simulink model "INS"  (R2022b)
settings: configuration reference "ins_config" (kept outside this file)
values from neighbouring files (symbols this model uses):
  INS_EXPORT = Simulink.Parameter(INS_EXPORT_VALUE)    [ins_model_init.m]
  INS_PARAM = Simulink.Parameter(INS_PARAM_VALUE)    [ins_model_init.m]
undefined symbols (not defined in the file or in its folder): DiscIntNeverNeededParam, INS_CONST, INS_EXPORT_VALUE
libraries: simulink x116, FMT_Model_Lib x35
(part 5 of 5)

== system INS/Data_Fusion/Rotation_Filter/AHRS/Correct/Attitude_Correction/Attitude_Correct/Acc_Estimator/Measure_Acc/GPS_Meas_Acc ==
  reset : Inport
  gps_vel_O_mPs : Inport  Port=2
  Enable : EnablePort  StatesWhenEnabling=reset
  Integrator : DiscreteIntegrator  ExternalReset=level  SampleTime=-1  ICPrevOutput=DiscIntNeverNeededParam  ICPrevScaledInput=DiscIntNeverNeededParam
  Integrator1 : DiscreteIntegrator  ExternalReset=level  InitialConditionSource=external  SampleTime=-1  ICPrevOutput=DiscIntNeverNeededParam  ICPrevScaledInput=DiscIntNeverNeededParam
  Sum : Sum  Inputs=|++
  Sum1 : Sum  Inputs=|+-
  gain : Gain  Gain=2*zeta*fc
  gain1 : Gain  Gain=fc^2
  gps_acc_O_mPs2 : Outport  VectorParamsAs1DForOutWhenUnconnected=off
  wires:
  Integrator1/1 -> Sum1/2
  Integrator/1 -> gps_acc_O_mPs2/1, Sum/2
  reset/1 -> Integrator1/2, Integrator/2
  gain/1 -> Sum/1
  Sum1/1 -> gain/1, gain1/1
  Sum/1 -> Integrator1/1
  gps_vel_O_mPs/1 -> Sum1/1, Integrator1/3
  gain1/1 -> Integrator/1

== system INS/Data_Fusion/Rotation_Filter/AHRS/Correct/Attitude_Correction/Attitude_Correct/Acc_Estimator/Measure_Acc/Valid_Check ==
  Sensor_Data : Inport
  Bus Selector : BusSelector  OutputSignals=GPS_Data.GPS_valid,GPS_Data.spd_quality
  Logical Operator1 : Logic  AllPortsSameDT=off  OutDataTypeStr=boolean
  Relay : Relay  OnSwitchValue=0.2  OffSwitchValue=0.1
  gps_meas_acc_valid : Outport  VectorParamsAs1DForOutWhenUnconnected=off
  wires:
  Sensor_Data/1 -> Bus Selector/1
  Logical Operator1/1 -> gps_meas_acc_valid/1
  Bus Selector/1 -> Logical Operator1/1  "<GPS_valid>"
  Relay/1 -> Logical Operator1/2
  Bus Selector/2 -> Relay/1  "<spd_quality>"

== system INS/Data_Fusion/Translation_Filter/CF/Bus_Constructor/Bus_Select/WGS84_Position/WGS84_Position/safe_divide/Zero_Value_Exclusion ==
  u : Inport
  Abs : Abs  SaturateOnIntegerOverflow=off
  Constant : Constant
  Product : Product  RndMeth=Zero
  Saturation : Saturate  UpperLimit=10e7  LowerLimit=1e-6
  Sign : Signum
  Switch : Switch  Criteria=u2 ~= 0  SaturateOnIntegerOverflow=off  InputSameDT=off
  y : Outport  VectorParamsAs1DForOutWhenUnconnected=off
  wires:
  u/1 -> Abs/1, Sign/1
  Abs/1 -> Saturation/1
  Saturation/1 -> Product/1
  Sign/1 -> Switch/2, Switch/1
  Product/1 -> y/1
  Switch/1 -> Product/2
  Constant/1 -> Switch/3

== system INS/Data_Fusion/Translation_Filter/CF/Horizontal_Filter/Correct/GPS Correct/GPS_Correct/Measurement/Bias_Estimation ==
  TF_Data : Inport
  X : Inport  Port=2
  xy_meas_m : Inport  Port=3
  Bias : Subsystem
  Sum1 : Sum  Inputs=|++
  bias_update : Outport  VectorParamsAs1DForOutWhenUnconnected=off
  xy_O_m : Outport  Port=2  VectorParamsAs1DForOutWhenUnconnected=off
  wires:
  TF_Data/1 -> Bias/3(TF_Data)
  X/1 -> Bias/2(X)
  Sum1/1 -> xy_O_m/1
  Bias/1(bias) -> Sum1/2
  xy_meas_m/1 -> Sum1/1, Bias/1(xy_meas_m)  "gps_xy_m"
  Bias/2(bias_update) -> bias_update/1

== system INS/Data_Fusion/Translation_Filter/CF/Horizontal_Filter/Predict/Propagate/States_Init/Pos_Init/GPS_Pos_Init ==
  TF_Data : Inport
  Enable : EnablePort
  Bus Selector : BusSelector  OutputSignals=Sensor_Meas.GPS_Meas.lat_rad,Sensor_Meas.GPS_Meas.lon_rad,TF_Control.WGS84_Ref.WGS84_pos_ref.lat_0_rad,TF_Control.WGS84_Ref.WGS84_pos_ref.lon_0_rad,TF_Control.WGS84_Ref.WGS84_derivatives_ref.dx_dlat_0,TF_Control.WGS84_Ref.WGS84_derivatives_ref.dy_dlon_0
  Data Type Conversion : DataTypeConversion  OutDataTypeStr=single  SaturateOnIntegerOverflow=off  RndMeth=Floor
  Multiply : Product
  Mux1 : Mux  Inputs=2
  Mux2 : Mux  Inputs=2
  Mux3 : Mux  Inputs=2
  Sum : Sum  Inputs=|+-
  X_0 : Outport  VectorParamsAs1DForOutWhenUnconnected=off
  wires:
  Data Type Conversion/1 -> X_0/1
  Bus Selector/1 -> Mux1/1  "<lat_rad>"
  Mux3/1 -> Multiply/2
  Bus Selector/3 -> Mux2/1  "<lat_0_rad>"
  Bus Selector/4 -> Mux2/2  "<lon_0_rad>"
  Mux2/1 -> Sum/2
  Bus Selector/6 -> Mux3/2  "<dy_dlon_0>"
  Mux1/1 -> Sum/1
  Sum/1 -> Multiply/1
  Bus Selector/5 -> Mux3/1  "<dx_dlat_0>"
  Bus Selector/2 -> Mux1/2  "<lon_rad>"
  TF_Data/1 -> Bus Selector/1
  Multiply/1 -> Data Type Conversion/1  "xy_R_m"

== system INS/Data_Fusion/Translation_Filter/CF/Horizontal_Filter/Predict/Propagate/States_Init/Vel_Init/GPS_Vel_Init ==
  Processed_Data : Inport
  Enable : EnablePort
  Bus Selector : BusSelector  OutputSignals=Sensor_Meas.GPS_Meas.vn_mPs,Sensor_Meas.GPS_Meas.ve_mPs
  Mux : Mux  Inputs=2
  Reshape : Reshape  OutputDimensionality=Customize  OutputDimensions=[2,1]
  Vel_NE_0 : Outport  VectorParamsAs1DForOutWhenUnconnected=off
  wires:
  Mux/1 -> Reshape/1
  Reshape/1 -> Vel_NE_0/1
  Bus Selector/2 -> Mux/2  "<ve_mPs>"
  Bus Selector/1 -> Mux/1  "<vn_mPs>"
  Processed_Data/1 -> Bus Selector/1

== system INS/Data_Fusion/Translation_Filter/CF/Horizontal_Filter/Predict/Propagate/States_Init/Vel_Init/OptFlow_Vel_Init ==
  Processed_Data : Inport
  Enable : EnablePort
  Bus Selector : BusSelector  OutputSignals=Sensor_Meas.OptFlow_Meas.vx_O_mPs,Sensor_Meas.OptFlow_Meas.vy_O_mPs
  Mux : Mux  Inputs=2
  Reshape : Reshape  OutputDimensionality=Column vector (2-D)  OutputDimensions=[2,1]
  Vel_NE_0 : Outport  VectorParamsAs1DForOutWhenUnconnected=off
  wires:
  Processed_Data/1 -> Bus Selector/1
  Bus Selector/1 -> Mux/1  "<vx_O_mPs>"
  Bus Selector/2 -> Mux/2  "<vy_O_mPs>"
  Reshape/1 -> Vel_NE_0/1
  Mux/1 -> Reshape/1

== system INS/Data_Fusion/Translation_Filter/CF/Verticle_Filter/Correct/Baro_Correct/Baro_Correct/Measurement/Bias_Estimation ==
  h_m : Inport
  TF_Data : Inport  Port=2
  X : Inport  Port=3
  Bias : Subsystem
  Bus Selector1 : BusSelector  OutputSignals=Sensor_Enable.vert_select.baro_enable
  Delay : Delay  DelayLength=1
  Detect Increase : simulink/Logic and Bit Operations/Detect Increase  vinit=0  OutDataTypeStr=boolean
  Selector : Selector  InputPortWidth=3  IndexOptions=Index vector (dialog)  Indices=1  OutputSizes=1
  Switch : Switch  Criteria=u2 > Threshold  OutDataTypeStr=single  SaturateOnIntegerOverflow=off  InputSameDT=off
  bias : Outport  VectorParamsAs1DForOutWhenUnconnected=off
  bias_update : Outport  Port=2  VectorParamsAs1DForOutWhenUnconnected=off
  wires:
  Delay/1 -> Switch/3
  X/1 -> Selector/1
  Bias/1(bias) -> Switch/1
  Switch/1 -> Delay/1, bias/1  "baro_alt_bias"
  Selector/1 -> Bias/1(height_est_m)
  h_m/1 -> Bias/2(height_meas_m)
  Bus Selector1/1 -> Detect Increase/1  "<baro_enable>"
  TF_Data/1 -> Bus Selector1/1
  Detect Increase/1 -> bias_update/1, Switch/2  "baro_bias_update"

== system INS/Data_Fusion/Translation_Filter/CF/Verticle_Filter/Correct/GPS_Correct/GPS_Correct/Measurement/Bias_Estimation ==
  h_m : Inport
  X : Inport  Port=2
  TF_Data : Inport  Port=3
  Bias : Subsystem
  Bus Selector1 : BusSelector  OutputSignals=Sensor_Enable.vert_select.gps_enable
  Detect Increase : simulink/Logic and Bit Operations/Detect Increase  vinit=0.0  OutDataTypeStr=boolean
  Memory : Memory
  Selector : Selector  InputPortWidth=3  IndexOptions=Index vector (dialog)  Indices=1  OutputSizes=1
  Switch : Switch  Criteria=u2 > Threshold  OutDataTypeStr=single  SaturateOnIntegerOverflow=off  InputSameDT=off
  bias : Outport  VectorParamsAs1DForOutWhenUnconnected=off
  bias_update : Outport  Port=2  VectorParamsAs1DForOutWhenUnconnected=off
  wires:
  Memory/1 -> Switch/3
  X/1 -> Selector/1
  Bias/1(bias) -> Switch/1
  Switch/1 -> Memory/1, bias/1  "gps_height_bias"
  Selector/1 -> Bias/1(h_est_m)  "h_est_m1"
  Bus Selector1/1 -> Detect Increase/1  "<gps_enable>"
  Detect Increase/1 -> bias_update/1, Switch/2
  TF_Data/1 -> Bus Selector1/1
  h_m/1 -> Bias/2(h_meas_m)  "gps_h_meas"

== system INS/Data_Fusion/Translation_Filter/CF/Verticle_Filter/Correct/Rf_Correct/Rangefinder_Correct/Measurement/Bias_Estimation ==
  h_m : Inport
  X : Inport  Port=2
  TF_Data : Inport  Port=3
  Bias : Subsystem
  Bus Selector1 : BusSelector  OutputSignals=Sensor_Enable.vert_select.rf_enable
  Detect Increase : simulink/Logic and Bit Operations/Detect Increase  vinit=0.0  OutDataTypeStr=boolean
  Detect_Jump_Signal : Subsystem
  Logical Operator : Logic  Operator=OR  AllPortsSameDT=off  OutDataTypeStr=boolean
  Memory : Memory
  Selector : Selector  InputPortWidth=3  IndexOptions=Index vector (dialog)  Indices=1  OutputSizes=1
  Switch : Switch  Criteria=u2 > Threshold  OutDataTypeStr=single  SaturateOnIntegerOverflow=off  InputSameDT=off
  bias : Outport  VectorParamsAs1DForOutWhenUnconnected=off
  bias_update : Outport  Port=2  VectorParamsAs1DForOutWhenUnconnected=off
  wires:
  Memory/1 -> Switch/3
  X/1 -> Selector/1
  Bias/1(bias) -> Switch/1
  Switch/1 -> Memory/1, bias/1  "rf_height_bias"
  Selector/1 -> Bias/1(h_est_m)  "rf_h_est_m"
  Bus Selector1/1 -> Detect Increase/1  "<rf_enable>"
  Logical Operator/1 -> Switch/2, bias_update/1
  TF_Data/1 -> Bus Selector1/1
  h_m/1 -> Detect_Jump_Signal/1(h_meas_m), Bias/2(h_meas_m)  "rf_h_meas"
  Detect Increase/1 -> Logical Operator/1
  Detect_Jump_Signal/1(update) -> Logical Operator/2

== system INS/Data_Fusion/Translation_Filter/CF/Verticle_Filter/Predict/Propagate/States_Init/Height_Init/Baro_Reference_Height ==
  TF_Data : Inport
  Enable : EnablePort
  Bus Selector : BusSelector  OutputSignals=Sensor_Meas.Baro_Meas.h_R_m
  Data Type Conversion : DataTypeConversion  OutDataTypeStr=single  SaturateOnIntegerOverflow=off  RndMeth=Floor
  h_R_m : Outport  VectorParamsAs1DForOutWhenUnconnected=off
  wires:
  Data Type Conversion/1 -> h_R_m/1
  Bus Selector/1 -> Data Type Conversion/1  "<h_R_m>"
  TF_Data/1 -> Bus Selector/1

== system INS/Data_Fusion/Translation_Filter/CF/Verticle_Filter/Predict/Propagate/States_Init/Height_Init/GPS_Reference_Height ==
  TF_Data : Inport
  Enable : EnablePort
  Bus Selector : BusSelector  OutputSignals=Sensor_Meas.GPS_Meas.h_m,TF_Control.WGS84_Ref.WGS84_pos_ref.h_0_m
  Data Type Conversion : DataTypeConversion  OutDataTypeStr=single  SaturateOnIntegerOverflow=off  RndMeth=Floor
  Sum : Sum  Inputs=|+-
  h_R_m : Outport  VectorParamsAs1DForOutWhenUnconnected=off
  wires:
  Data Type Conversion/1 -> h_R_m/1
  Bus Selector/2 -> Sum/2  "<h_0_m>"
  Bus Selector/1 -> Sum/1  "<h_m>"
  TF_Data/1 -> Bus Selector/1
  Sum/1 -> Data Type Conversion/1  "h_R_m"

== system INS/Data_Fusion/Translation_Filter/CF/Verticle_Filter/Predict/Propagate/States_Init/Height_Init/Rf_Reference_Height ==
  TF_Data : Inport
  Enable : EnablePort
  Bus Selector : BusSelector  OutputSignals=Sensor_Meas.Rf_Meas.h_AGL_m
  Data Type Conversion : DataTypeConversion  OutDataTypeStr=single  SaturateOnIntegerOverflow=off  RndMeth=Floor
  h_R_m : Outport  VectorParamsAs1DForOutWhenUnconnected=off
  wires:
  TF_Data/1 -> Bus Selector/1
  Bus Selector/1 -> Data Type Conversion/1  "<h_AGL_m>"
  Data Type Conversion/1 -> h_R_m/1

== system INS/Data_Fusion/Translation_Filter/CF/Verticle_Filter/Predict/Propagate/States_Init/Velocity_Init/Baro_Velocity ==
  TF_Data : Inport
  Enable : EnablePort
  Constant : Constant  Value=0  OutDataTypeStr=single
  Terminator : Terminator
  vel_D_mPs : Outport  VectorParamsAs1DForOutWhenUnconnected=off
  wires:
  Constant/1 -> vel_D_mPs/1
  TF_Data/1 -> Terminator/1

== system INS/Data_Fusion/Translation_Filter/CF/Verticle_Filter/Predict/Propagate/States_Init/Velocity_Init/GPS_Velocity ==
  TF_Data : Inport
  Enable : EnablePort
  Bus Selector : BusSelector  OutputSignals=Sensor_Meas.GPS_Meas.vd_mPs
  Data Type Conversion : DataTypeConversion  OutDataTypeStr=single  SaturateOnIntegerOverflow=off  RndMeth=Floor
  vel_D_mPs : Outport  VectorParamsAs1DForOutWhenUnconnected=off
  wires:
  Data Type Conversion/1 -> vel_D_mPs/1
  Bus Selector/1 -> Data Type Conversion/1  "<vd_mPs>"
  TF_Data/1 -> Bus Selector/1

== system INS/Data_Fusion/Translation_Filter/CF/Verticle_Filter/Predict/Propagate/States_Init/Velocity_Init/Rf_Velocity ==
  TF_Data : Inport
  Enable : EnablePort
  Constant : Constant  Value=0  OutDataTypeStr=single
  Terminator : Terminator
  vel_D_mPs : Outport  VectorParamsAs1DForOutWhenUnconnected=off
  wires:
  Constant/1 -> vel_D_mPs/1
  TF_Data/1 -> Terminator/1

== system INS/Data_Fusion/Translation_Filter/CF/Horizontal_Filter/Correct/GPS Correct/GPS_Correct/Measurement/Bias_Estimation/Bias ==
  xy_meas_m : Inport
  X : Inport  Port=2
  TF_Data : Inport  Port=3
  Bias_Update : Subsystem
  Bus Selector1 : BusSelector  OutputSignals=Sensor_Enable.horizon_select.gps_enable
  Detect Increase : simulink/Logic and Bit Operations/Detect Increase  vinit=0.0  OutDataTypeStr=boolean
  Memory : Memory  InitialCondition=[0;0]
  Selector : Selector  InputPortWidth=6  IndexOptions=Index vector (dialog)  Indices=[1 2]  OutputSizes=1
  Switch : Switch  Criteria=u2 > Threshold  OutDataTypeStr=single  SaturateOnIntegerOverflow=off  InputSameDT=off
  bias : Outport  VectorParamsAs1DForOutWhenUnconnected=off
  bias_update : Outport  Port=2  VectorParamsAs1DForOutWhenUnconnected=off
  wires:
  xy_meas_m/1 -> Bias_Update/2(xy_meas_m)
  TF_Data/1 -> Bus Selector1/1
  Detect Increase/1 -> bias_update/1, Switch/2
  Bus Selector1/1 -> Detect Increase/1  "<gps_enable>"
  Selector/1 -> Bias_Update/1(xy_est_m)  "gps_xy_est"
  Switch/1 -> bias/1, Memory/1  "gps_pos_bias"
  Bias_Update/1(bias) -> Switch/1
  X/1 -> Selector/1
  Memory/1 -> Switch/3

== system INS/Data_Fusion/Translation_Filter/CF/Verticle_Filter/Correct/Baro_Correct/Baro_Correct/Measurement/Bias_Estimation/Bias ==
  height_est_m : Inport
  height_meas_m : Inport  Port=2
  Sum : Sum  Inputs=+-|
  bias : Outport  VectorParamsAs1DForOutWhenUnconnected=off
  wires:
  Sum/1 -> bias/1
  height_meas_m/1 -> Sum/2  "height_meas_m"
  height_est_m/1 -> Sum/1  "height_est_m"

== system INS/Data_Fusion/Translation_Filter/CF/Verticle_Filter/Correct/GPS_Correct/GPS_Correct/Measurement/Bias_Estimation/Bias ==
  h_est_m : Inport
  h_meas_m : Inport  Port=2
  Sum : Sum  Inputs=+-|
  bias : Outport  VectorParamsAs1DForOutWhenUnconnected=off
  wires:
  Sum/1 -> bias/1
  h_meas_m/1 -> Sum/2
  h_est_m/1 -> Sum/1

== system INS/Data_Fusion/Translation_Filter/CF/Verticle_Filter/Correct/Rf_Correct/Rangefinder_Correct/Measurement/Bias_Estimation/Bias ==
  h_est_m : Inport
  h_meas_m : Inport  Port=2
  Sum : Sum  Inputs=+-|
  bias : Outport  VectorParamsAs1DForOutWhenUnconnected=off
  wires:
  Sum/1 -> bias/1
  h_meas_m/1 -> Sum/2
  h_est_m/1 -> Sum/1

== system INS/Data_Fusion/Translation_Filter/CF/Verticle_Filter/Correct/Rf_Correct/Rangefinder_Correct/Measurement/Bias_Estimation/Detect_Jump_Signal ==
  h_meas_m : Inport
  1/dT : Gain  Gain=100
  Abs : Abs  SaturateOnIntegerOverflow=off
  Compare To Constant : simulink/Logic and Bit Operations/Compare To Constant  relop=>  const=5  OutDataTypeStr=boolean
  Delay : Delay  DelayLength=1
  Sum : Sum  Inputs=|+-
  update : Outport  VectorParamsAs1DForOutWhenUnconnected=off
  wires:
  h_meas_m/1 -> Sum/1, Delay/1
  Delay/1 -> Sum/2
  Sum/1 -> 1/dT/1
  1/dT/1 -> Abs/1
  Abs/1 -> Compare To Constant/1
  Compare To Constant/1 -> update/1

== system INS/Data_Fusion/Translation_Filter/CF/Horizontal_Filter/Correct/GPS Correct/GPS_Correct/Measurement/Bias_Estimation/Bias/Bias_Update ==
  xy_est_m : Inport
  xy_meas_m : Inport  Port=2
  Sum : Sum  Inputs=+-|
  bias : Outport  VectorParamsAs1DForOutWhenUnconnected=off
  wires:
  xy_est_m/1 -> Sum/1
  xy_meas_m/1 -> Sum/2
  Sum/1 -> bias/1
